simulink model "path_following_control"  (R2021a)
settings: Solver=VariableStepAuto  StartTime=0.0  StopTime=10.0  RelTol=1e-3
values from neighbouring files (symbols this model uses):
  Cf = 155494.663    [Combined_Control_Model.m]
  Cr = 1554494.663    [Combined_Control_Model.m]
  Iz = 1436.24    [Combined_Control_Model.m]
  lf = 1.165    [Combined_Control_Model.m]
  lr = 1.165    [Combined_Control_Model.m]
  m = 1140    [Combined_Control_Model.m]
  md = get_curvature(Vx, yaw_rate_pose, tRef)    [Combined_Control_Model.m]
  Ts = 0.1    [Combined_Control_Model.m]
  v0_ego = 25    [Combined_Control_Model.m]
  v0_lead = 25    [Combined_Control_Model.m]
  x0_ego = 10    [Combined_Control_Model.m]
  x0_lead = 50    [Combined_Control_Model.m]
libraries: mpcadaslib x1
settings Model: Creator=User  LastModifiedBy=User

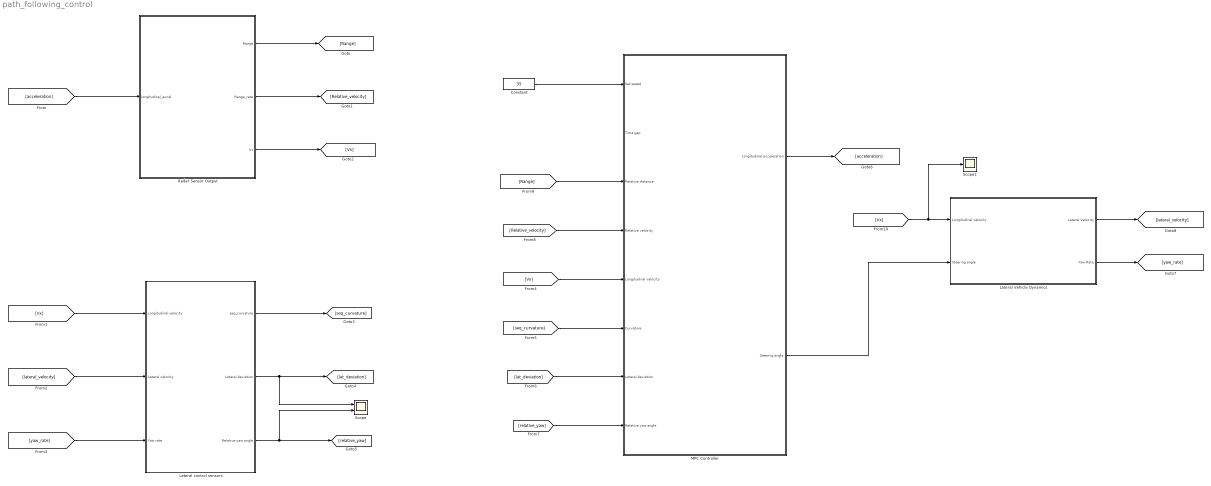
== system path_following_control ==
  Constant : Constant  Value=35
  Lateral Vehicle Dynamics : Subsystem
  Lateral control sensors : Subsystem
  MPC Controller : Subsystem
  Radar Sensor Output : Subsystem
  Scope : Scope  NumInputPorts=2
  Scope1 : Scope
  wires:
  Radar Sensor Output/1(Range) -> [Range]
  Radar Sensor Output/2(Range_rate) -> [Relative_velocity]
  Radar Sensor Output/3(Vx) -> [Vx]
  Lateral control sensors/1(seq_curvature) -> [seq_curvature]
  Lateral control sensors/2(Lateral deviation) -> Scope/1, [lat_deviation]
  Lateral control sensors/3(Relative yaw angle) -> Scope/2, [relative_yaw]
  [acceleration] -> Radar Sensor Output/1(longitudinal_accel)
  [yaw_rate] -> Lateral control sensors/3(Yaw rate)
  [lateral_velocity] -> Lateral control sensors/2(Lateral velocity)
  [Vx] -> Lateral control sensors/1(Longitudinal velocity)
  Constant/1 -> MPC Controller/1(Set speed)
  [Vx] -> MPC Controller/5(Longitudinal velocity)
  [seq_curvature] -> MPC Controller/6(Curvature)
  [lat_deviation] -> MPC Controller/7(Lateral deviation)
  [relative_yaw] -> MPC Controller/8(Relative yaw angle)
  [Relative_velocity] -> MPC Controller/4(Relative velocity)
  [Range] -> MPC Controller/3(Relative distance)
  MPC Controller/1(Longitudinal acceleration) -> [acceleration]
  [Vx] -> Scope1/1, Lateral Vehicle Dynamics/1(Longitudinal velocity)
  MPC Controller/2(Steering angle) -> Lateral Vehicle Dynamics/2(Steering angle)
  Lateral Vehicle Dynamics/1(Lateral Velocity) -> [lateral_velocity]
  Lateral Vehicle Dynamics/2(Yaw Rate) -> [yaw_rate]

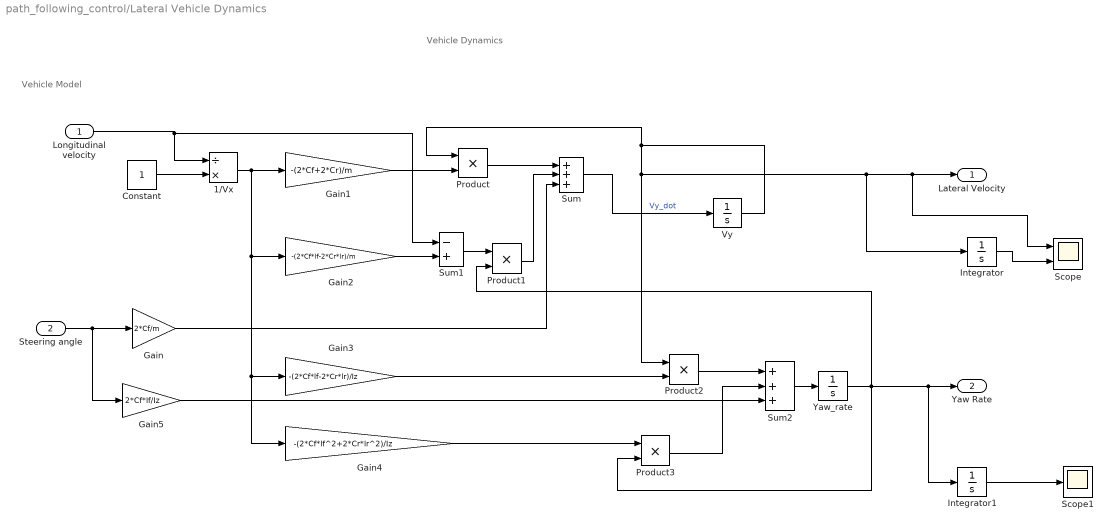
== system path_following_control/Lateral Vehicle Dynamics ==
  note: Vehicle Model
  note: Vehicle Dynamics
  Longitudinal velocity : Inport
  Steering angle : Inport  Port=2
  1/Vx : Product  Inputs=/*
  Constant : Constant
  Gain : Gain  Gain=2*Cf/m
  Gain1 : Gain  Gain=-(2*Cf+2*Cr)/m
  Gain2 : Gain  Gain=-(2*Cf*lf-2*Cr*lr)/m
  Gain3 : Gain  Gain=-(2*Cf*lf-2*Cr*lr)/Iz
  Gain4 : Gain  Gain=-(2*Cf*lf^2+2*Cr*lr^2)/Iz
  Gain5 : Gain  Gain=2*Cf*lf/Iz
  Integrator : Integrator
  Integrator1 : Integrator
  Product{,1..3} (4 alike) : Product
  Scope : Scope  NumInputPorts=2
  Scope1 : Scope
  Sum : Sum  Inputs=+++
  Sum1 : Sum  Inputs=-+
  Sum2 : Sum  Inputs=+++
  Vy : Integrator
  "Yaw_rate " : Integrator
  Lateral Velocity : Outport  VectorParamsAs1DForOutWhenUnconnected=off
  Yaw Rate : Outport  Port=2  VectorParamsAs1DForOutWhenUnconnected=off
  wires:
  Sum2/1 -> "Yaw_rate "/1
  Gain2/1 -> Sum1/2
  Gain4/1 -> Product3/1
  Constant/1 -> 1/Vx/2
  Gain3/1 -> Product2/2
  1/Vx/1 -> Gain4/1, Gain3/1, Gain2/1, Gain1/1
  Product2/1 -> Sum2/1
  Product3/1 -> Sum2/2
  Gain5/1 -> Sum2/3
  Sum1/1 -> Product1/1
  "Yaw_rate "/1 -> Product3/2, Integrator1/1, Yaw Rate/1, Product1/2
  Gain/1 -> Sum/3
  Steering angle/1 -> Gain/1, Gain5/1
  Gain1/1 -> Product/2
  Product/1 -> Sum/1
  Vy/1 -> Product/1, Integrator/1, Scope/1, Lateral Velocity/1, Product2/1
  Sum/1 -> Vy/1  "Vy_dot"
  Longitudinal velocity/1 -> Sum1/1, 1/Vx/1
  Product1/1 -> Sum/2
  Integrator/1 -> Scope/2
  Integrator1/1 -> Scope1/1

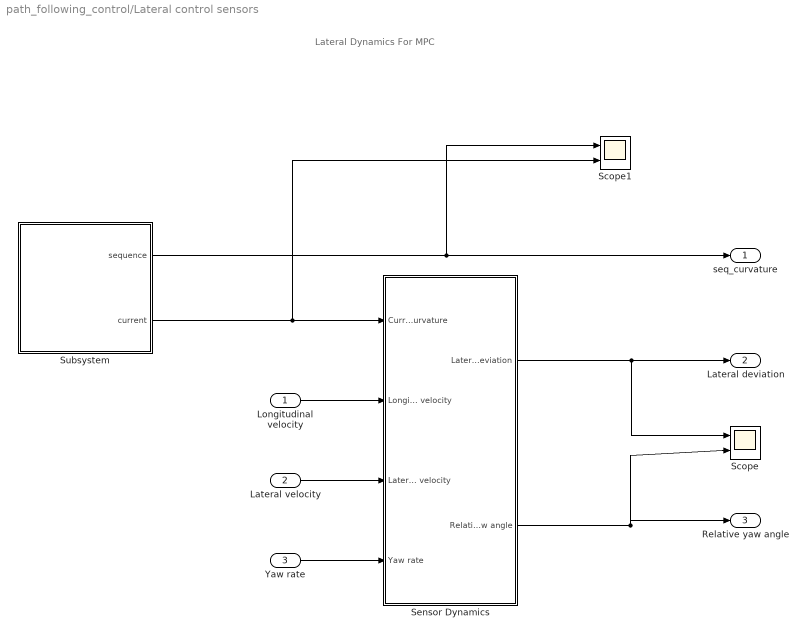
== system path_following_control/Lateral control sensors ==
  note: Lateral Dynamics For MPC
  Longitudinal velocity : Inport
  Lateral velocity : Inport  Port=2
  Yaw rate : Inport  Port=3
  Scope : Scope  NumInputPorts=2
  Scope1 : Scope  NumInputPorts=2
  Sensor Dynamics : Subsystem
  Subsystem : Subsystem  mask{signal=md, ts=Ts, steps=10}
      mask prompts: signal "Signal name"; ts "Sampling time"; steps "Number of previewing steps"
      mask init:
      | ts = evalin('base',get_param(gcbh,'ts'));
      | signal = evalin('base',get_param(gcbh,'signal'));
      | steps = evalin('base',get_param(gcbh,'steps'));
      | data = mpc_previewer_maskinit(signal,ts);
      mask Display:
      | fprintf('Future\nsample\nextractor');
      | port_label('output', 1, 'seq')
      | port_label('output', 2, '@t')
  seq_curvature : Outport
  Lateral deviation : Outport  Port=2
  Relative yaw angle : Outport  Port=3
  wires:
  Lateral velocity/1 -> Sensor Dynamics/3(Lateral velocity)
  Subsystem/2(current) -> Sensor Dynamics/1(Current curvature), Scope1/2
  Yaw rate/1 -> Sensor Dynamics/4(Yaw rate)
  Sensor Dynamics/1(Lateral deviation) -> Scope/1, Lateral deviation/1
  Sensor Dynamics/2(Relative yaw angle) -> Scope/2, Relative yaw angle/1
  Subsystem/1(sequence) -> Scope1/1, seq_curvature/1
  Longitudinal velocity/1 -> Sensor Dynamics/2(Longitudinal velocity)

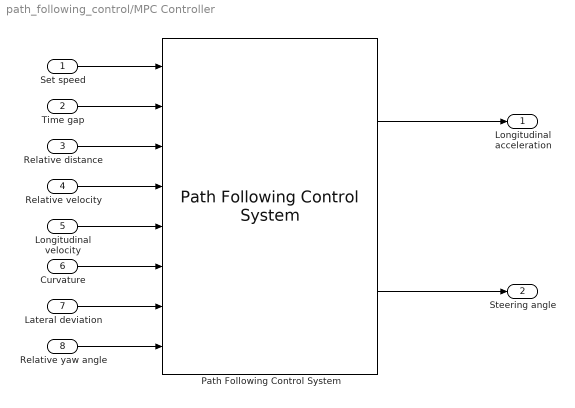
== system path_following_control/MPC Controller ==
  Set speed : Inport
  Time gap : Inport  Port=2
  Relative distance : Inport  Port=3
  Relative velocity : Inport  Port=4
  Longitudinal velocity : Inport  Port=5
  Curvature : Inport  Port=6
  Lateral deviation : Inport  Port=7
  Relative yaw angle : Inport  Port=8
  Path Following Control System : mpcadaslib/Path Following Control System  VariantControl=Variant2  ModelType=Use vehicle parameters  VehicleMass=m  VehicleYawInertia=Iz  LengthToFront=lf  LengthToRear=lr  FrontTireStiffness=Cf  RearTireStiffness=Cr  AccelTimeConstant=tau  EgoModelMatrixA=[-2,zeros(1,3);1,zeros(1,3);zeros(1,2),-4.4021,-12.4603;zeros(1,2),1.3913,-5.1868]  EgoModelMatrixB=[2,zeros(1,3);zeros(1,2),24.1270,15.8609]'  EgoModelMatrixC=[zeros(3,1),eye(3)]  InitialLongVel=v0_ego  TransportLag=0  spaceCtrl=on  DefaultSpacing=10  MinSteering=-0.5  umin_ext=off  MaxSteering=0.5  umax_ext=off  MinAcceleration=-3  amin_ext=off  MaxAcceleration=2  amax_ext=off  Ts=0.1  PredictionHorizon=PredictionHorizon  ControlHorizon=3  LongWeight=0.5  LateralWeight=1  AccelRateWeight=0.1  SteerRateWeight=0.1  suboptimal=off  maxiter=10  datatypeopt=double  optmode=off  trackmode=off
      settings: SourceProductBaseCode=MP
  Longitudinal acceleration : Outport
  Steering angle : Outport  Port=2
  wires:
  Set speed/1 -> Path Following Control System/1
  Relative distance/1 -> Path Following Control System/3
  Relative velocity/1 -> Path Following Control System/4
  Longitudinal velocity/1 -> Path Following Control System/5
  Curvature/1 -> Path Following Control System/6
  Lateral deviation/1 -> Path Following Control System/7
  Relative yaw angle/1 -> Path Following Control System/8
  Path Following Control System/2 -> Steering angle/1
  Path Following Control System/1 -> Longitudinal acceleration/1
  Time gap/1 -> Path Following Control System/2

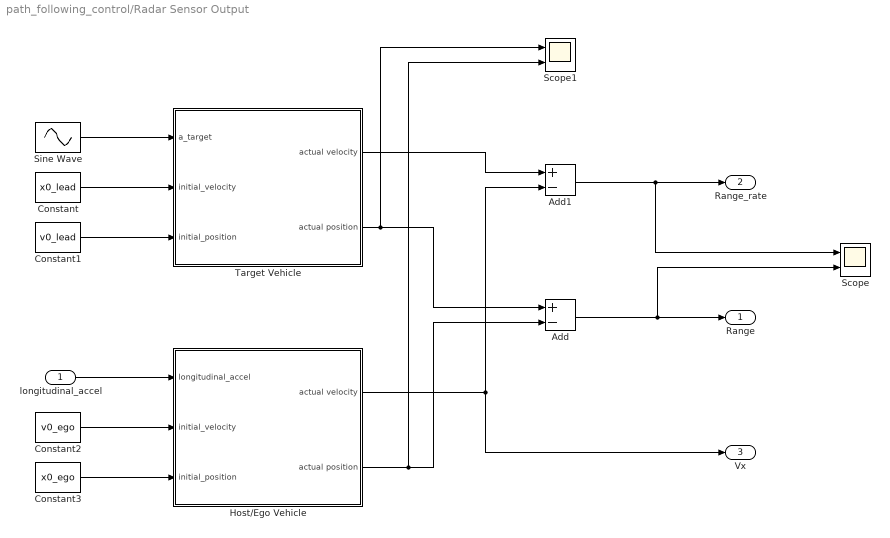
== system path_following_control/Radar Sensor Output ==
  longitudinal_accel : Inport
  Add : Sum  Inputs=+-
  Add1 : Sum  Inputs=+-
  Constant : Constant  Value=x0_lead
  Constant1 : Constant  Value=v0_lead
  Constant2 : Constant  Value=v0_ego
  Constant3 : Constant  Value=x0_ego
  Host/Ego Vehicle : Subsystem
  Scope : Scope  NumInputPorts=2
  Scope1 : Scope  NumInputPorts=2
  Sine Wave : Sin  Amplitude=0.6  Frequency=0.5  SampleTime=Ts
  Target Vehicle : Subsystem
  Range : Outport
  Range_rate : Outport  Port=2
  Vx : Outport  Port=3
  wires:
  Sine Wave/1 -> Target Vehicle/1(a_target)
  Constant1/1 -> Target Vehicle/3(initial_position)
  Constant/1 -> Target Vehicle/2(initial_velocity)
  Constant2/1 -> Host/Ego Vehicle/2(initial_velocity)
  Constant3/1 -> Host/Ego Vehicle/3(initial_position)
  longitudinal_accel/1 -> Host/Ego Vehicle/1(longitudinal_accel)
  Host/Ego Vehicle/2(actual position) -> Scope1/2, Add/2
  Target Vehicle/2(actual position) -> Scope1/1, Add/1
  Add/1 -> Scope/2, Range/1
  Add1/1 -> Scope/1, Range_rate/1
  Host/Ego Vehicle/1(actual velocity) -> Vx/1, Add1/2
  Target Vehicle/1(actual velocity) -> Add1/1

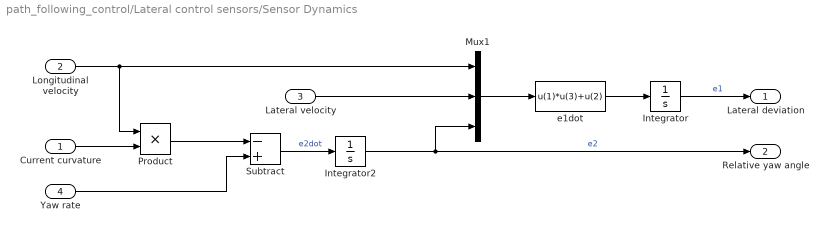
== system path_following_control/Lateral control sensors/Sensor Dynamics ==
  Current curvature : Inport
  Longitudinal velocity : Inport  Port=2
  Lateral velocity : Inport  Port=3
  Yaw rate : Inport  Port=4
  Integrator : Integrator
  Integrator2 : Integrator
  Mux1 : Mux  Inputs=[1 1 1]
  Product : Product
  Subtract : Sum  Inputs=-+
  e1dot : Fcn  Expr=u(1)*u(3)+u(2)
  Lateral deviation : Outport  VectorParamsAs1DForOutWhenUnconnected=off
  Relative yaw angle : Outport  Port=2  VectorParamsAs1DForOutWhenUnconnected=off
  wires:
  Current curvature/1 -> Product/2
  Integrator2/1 -> Mux1/3, Relative yaw angle/1  "e2"
  Mux1/1 -> e1dot/1
  e1dot/1 -> Integrator/1
  Longitudinal velocity/1 -> Product/1, Mux1/1
  Lateral velocity/1 -> Mux1/2
  Integrator/1 -> Lateral deviation/1  "e1"
  Product/1 -> Subtract/1
  Yaw rate/1 -> Subtract/2
  Subtract/1 -> Integrator2/1  "e2dot"

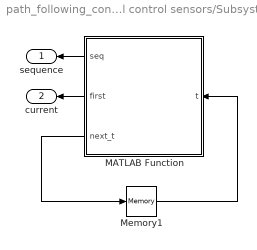
== system path_following_control/Lateral control sensors/Subsystem ==
  MATLAB Function : MATLAB Function  TreatAsAtomicUnit=on
  Memory1 : Memory  InheritSampleTime=on  LinearizeAsDelay=on
  sequence : Outport  VectorParamsAs1DForOutWhenUnconnected=off
  current : Outport  Port=2  VectorParamsAs1DForOutWhenUnconnected=off
  wires:
  MATLAB Function/2(first) -> current/1
  MATLAB Function/3(next_t) -> Memory1/1
  MATLAB Function/1(seq) -> sequence/1
  Memory1/1 -> MATLAB Function/1(t)

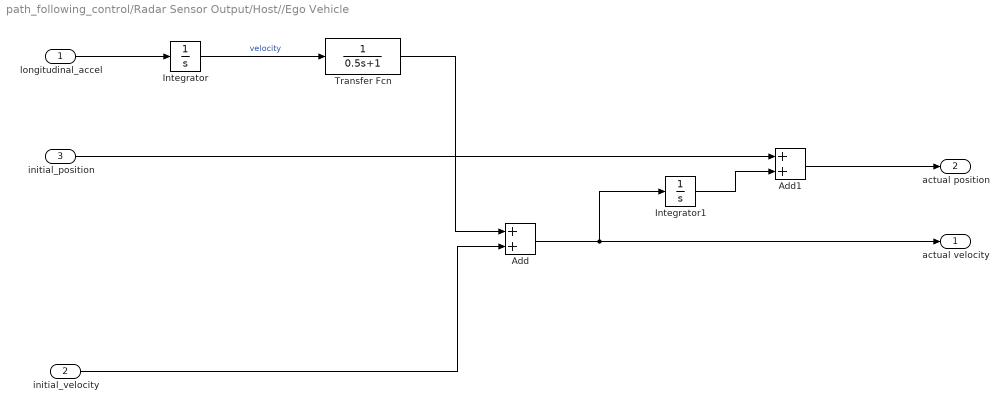
== system path_following_control/Radar Sensor Output/Host//Ego Vehicle ==
  longitudinal_accel : Inport
  initial_velocity : Inport  Port=2
  initial_position : Inport  Port=3
  Add : Sum
  Add1 : Sum
  Integrator : Integrator
  Integrator1 : Integrator
  Transfer Fcn : TransferFcn  Denominator=[0.5 1]
  actual velocity : Outport
  actual position : Outport  Port=2
  wires:
  Add1/1 -> actual position/1
  initial_position/1 -> Add1/1
  Integrator1/1 -> Add1/2
  Add/1 -> actual velocity/1, Integrator1/1
  initial_velocity/1 -> Add/2
  Transfer Fcn/1 -> Add/1
  Integrator/1 -> Transfer Fcn/1  "velocity"
  longitudinal_accel/1 -> Integrator/1

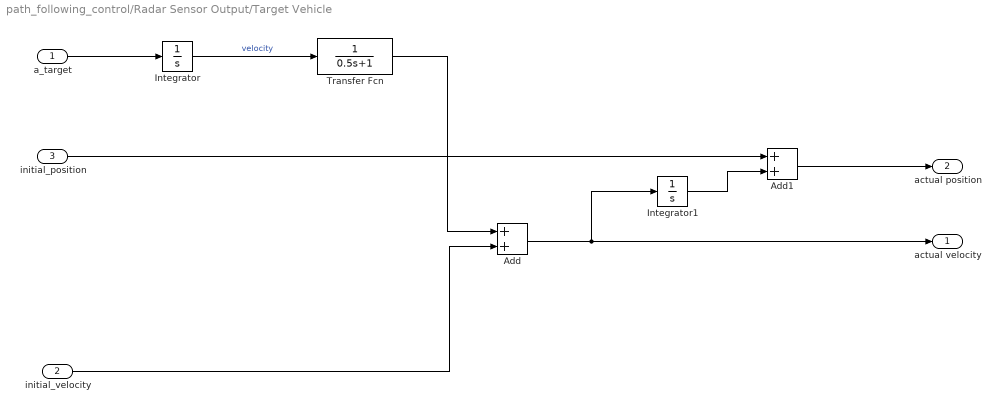
== system path_following_control/Radar Sensor Output/Target Vehicle ==
  a_target : Inport
  initial_velocity : Inport  Port=2
  initial_position : Inport  Port=3
  Add : Sum
  Add1 : Sum
  Integrator : Integrator
  Integrator1 : Integrator
  Transfer Fcn : TransferFcn  Denominator=[0.5 1]
  actual velocity : Outport
  actual position : Outport  Port=2
  wires:
  a_target/1 -> Integrator/1
  Integrator/1 -> Transfer Fcn/1  "velocity"
  Transfer Fcn/1 -> Add/1
  initial_velocity/1 -> Add/2
  Add/1 -> Integrator1/1, actual velocity/1
  Integrator1/1 -> Add1/2
  initial_position/1 -> Add1/1
  Add1/1 -> actual position/1

== matlab function path_following_control/Lateral control sensors/Subsystem/MATLAB Function ==
  settings: updateMethod=DISCRETE  sampleTime=ts
  data: data parameter; seq output; steps parameter; t input; first output; next_t output
function [seq,first,next_t] = fcn(data,steps,t)
%#codegen
[seq,first,next_t] = mpcblock_preview('md',data,steps,t);
